simulink model "quadcopter_control_1"  (R2024b)
settings: Solver=ode45  StartTime=0.0  StopTime=10  RelTol=1e-3
libraries: slpidlib x6
settings Model: Creator=lenovo x390  LastModifiedBy=lenovo x390

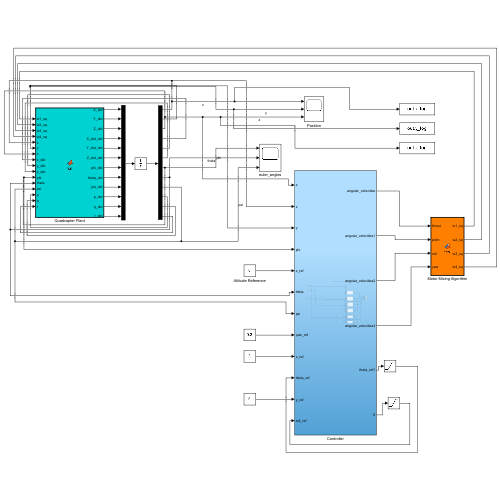
[thumbnail: Simulink's stored preview of the top-level diagram]
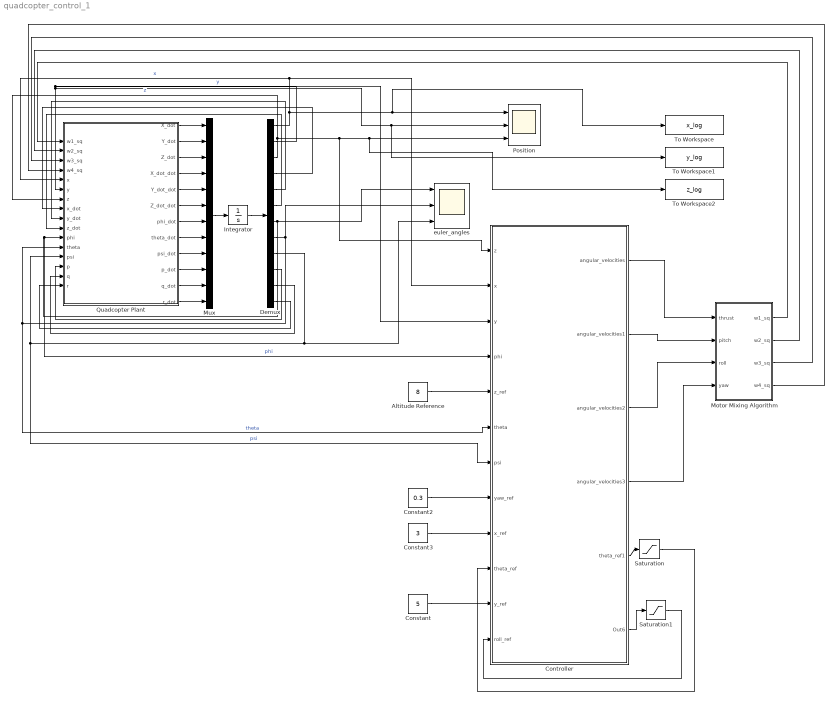
== system quadcopter_control_1 ==
  Altitude Reference : Constant  Value=8
  Constant : Constant  Value=5
  Constant2 : Constant  Value=0.3
  Constant3 : Constant  Value=3
  Controller : Subsystem
  Demux : Demux  Outputs=12
  Integrator : Integrator  InitialCondition=[0 0 1 0 0 0 0 0 0 0 0 0]
  Motor Mixing Algorithm : MATLAB Function  TreatAsAtomicUnit=on
  Mux : Mux  Inputs=12
  Position : Scope  NumInputPorts=3
  Quadcopter Plant : MATLAB Function  TreatAsAtomicUnit=on
  Saturation : Saturate
  Saturation1 : Saturate  UpperLimit=+0.3  LowerLimit=-0.3
  To Workspace : ToWorkspace  VariableName=x_log  SaveFormat=Timeseries  SampleTime=-1
  To Workspace1 : ToWorkspace  VariableName=y_log  SaveFormat=Timeseries  SampleTime=-1
  To Workspace2 : ToWorkspace  VariableName=z_log  SaveFormat=Timeseries  SampleTime=-1
  euler_angles : Scope  NumInputPorts=3
  wires:
  Quadcopter Plant/1(X_dot) -> Mux/1
  Quadcopter Plant/2(Y_dot) -> Mux/2
  Quadcopter Plant/3(Z_dot) -> Mux/3
  Quadcopter Plant/4(X_dot_dot) -> Mux/4
  Quadcopter Plant/5(Y_dot_dot) -> Mux/5
  Quadcopter Plant/6(Z_dot_dot) -> Mux/6
  Quadcopter Plant/7(phi_dot) -> Mux/7
  Quadcopter Plant/8(theta_dot) -> Mux/8
  Quadcopter Plant/9(psi_dot) -> Mux/9
  Quadcopter Plant/10(p_dot) -> Mux/10
  Quadcopter Plant/11(q_dot) -> Mux/11
  Quadcopter Plant/12(r_dot) -> Mux/12
  Mux/1 -> Integrator/1
  Integrator/1 -> Demux/1
  Demux/1 -> Quadcopter Plant/5(x), Controller/2(x), To Workspace/1, Position/1  "x"
  Demux/2 -> Quadcopter Plant/6(y), To Workspace1/1, Position/2, Controller/3(y)  "y"
  Demux/3 -> Quadcopter Plant/7(z), Controller/1(z), To Workspace2/1, Position/3  "z"
  Demux/4 -> Quadcopter Plant/8(x_dot)
  Demux/5 -> Quadcopter Plant/9(y_dot)
  Demux/6 -> Quadcopter Plant/10(z_dot)
  Demux/7 -> Controller/4(phi), Quadcopter Plant/11(phi), euler_angles/1  "phi"
  Demux/8 -> Controller/6(theta), Quadcopter Plant/12(theta), euler_angles/2  "theta"
  Demux/9 -> Controller/7(psi), Quadcopter Plant/13(psi), euler_angles/3  "psi"
  Demux/10 -> Quadcopter Plant/14(p)
  Demux/11 -> Quadcopter Plant/15(q)
  Demux/12 -> Quadcopter Plant/16(r)
  Motor Mixing Algorithm/1(w1_sq) -> Quadcopter Plant/1(w1_sq)
  Motor Mixing Algorithm/2(w2_sq) -> Quadcopter Plant/2(w2_sq)
  Motor Mixing Algorithm/3(w3_sq) -> Quadcopter Plant/3(w3_sq)
  Motor Mixing Algorithm/4(w4_sq) -> Quadcopter Plant/4(w4_sq)
  Altitude Reference/1 -> Controller/5(z_ref)
  Constant2/1 -> Controller/8(yaw_ref)
  Constant3/1 -> Controller/9(x_ref)
  Saturation/1 -> Controller/10(theta_ref)
  Constant/1 -> Controller/11(y_ref)
  Saturation1/1 -> Controller/12(roll_ref)
  Controller/1(angular_velocities) -> Motor Mixing Algorithm/1(thrust)
  Controller/2(angular_velocities1) -> Motor Mixing Algorithm/2(pitch)
  Controller/3(angular_velocities2) -> Motor Mixing Algorithm/3(roll)
  Controller/4(angular_velocities3) -> Motor Mixing Algorithm/4(yaw)
  Controller/5(theta_ref1) -> Saturation/1
  Controller/6(Out6) -> Saturation1/1

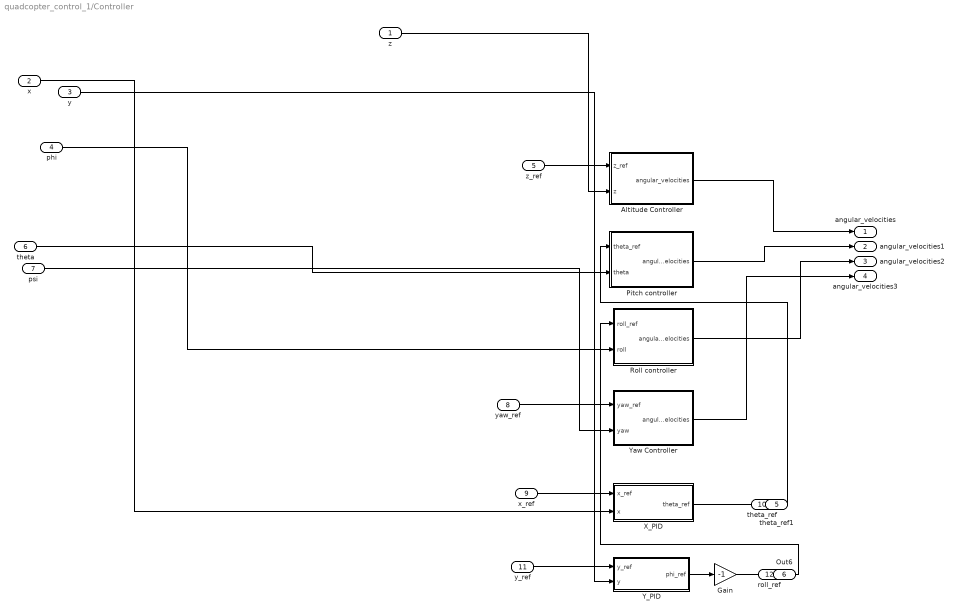
== system quadcopter_control_1/Controller ==
  z : Inport
  x : Inport  Port=2
  y : Inport  Port=3
  phi : Inport  Port=4
  z_ref : Inport  Port=5
  theta : Inport  Port=6
  psi : Inport  Port=7
  yaw_ref : Inport  Port=8
  x_ref : Inport  Port=9
  theta_ref : Inport  Port=10
  y_ref : Inport  Port=11
  roll_ref : Inport  Port=12
  Altitude Controller : Subsystem
  Gain : Gain  Gain=-1
  Pitch controller : Subsystem
  Roll controller : Subsystem
  X_PID : Subsystem
  Y_PID : Subsystem
  Yaw Controller : Subsystem
  angular_velocities : Outport
  angular_velocities1 : Outport  Port=2
  angular_velocities2 : Outport  Port=3
  angular_velocities3 : Outport  Port=4
  theta_ref1 : Outport  Port=5
  Out6 : Outport  Port=6
  wires:
  phi/1 -> Roll controller/2(roll)
  Pitch controller/1(angular_velocities) -> angular_velocities1/1
  theta/1 -> Pitch controller/2(theta)
  theta_ref/1 -> Pitch controller/1(theta_ref)
  Y_PID/1(phi_ref) -> Gain/1
  x/1 -> X_PID/2(x)
  Roll controller/1(angular_velocities) -> angular_velocities2/1
  Gain/1 -> Out6/1
  roll_ref/1 -> Roll controller/1(roll_ref)
  yaw_ref/1 -> Yaw Controller/1(yaw_ref)
  psi/1 -> Yaw Controller/2(yaw)
  x_ref/1 -> X_PID/1(x_ref)
  z_ref/1 -> Altitude Controller/1(z_ref)
  Yaw Controller/1(angular_velocities) -> angular_velocities3/1
  y/1 -> Y_PID/2(y)
  X_PID/1(theta_ref) -> theta_ref1/1
  z/1 -> Altitude Controller/2(z)
  Altitude Controller/1(angular_velocities) -> angular_velocities/1
  y_ref/1 -> Y_PID/1(y_ref)

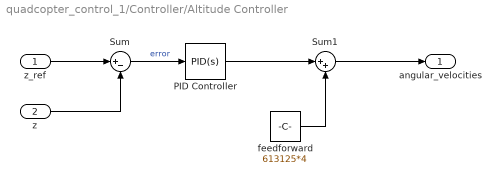
== system quadcopter_control_1/Controller/Altitude Controller ==
  z_ref : Inport
  z : Inport  Port=2
  PID Controller : slpidlib/PID Controller  Controller=PID  Form=Parallel  TimeDomain=Continuous-time  UseExternalTs=off  SampleTime=-1  IntegratorMethod=Forward Euler  FilterMethod=Forward Euler  ControllerParametersSource=internal  P=328860.941358092  I=45284.5767226925  UseKiTs=off  D=525153.531674945  UseExternalDerivativeSource=off  N=245.289249242135  UseFilter=on  TunerSelectOption=Transfer Function Based (PID Tuner App)  InitialConditionSource=internal  InitialConditionForIntegrator=0  InitialConditionForFilter=0  DifferentiatorICPrevScaledInput=0  ExternalReset=none  TrackingMode=off  Kt=1  LimitOutput=off  SatLimitsSource=internal  UpperSaturationLimit=inf  LowerSaturationLimit=-inf  LinearizeAsGain=on  AntiWindupMode=none  Kb=1  LimitIntegrator=off  UpperIntegratorSaturationLimit=inf  LowerIntegratorSaturationLimit=-inf  POutMin=[]  POutMax=[]  IOutMin=[]  IOutMax=[]  DOutMin=[]  DOutMax=[]  NOutMin=[]  NOutMax=[]  SumOutMin=[]  SumOutMax=[]  SaturationOutMin=[]  SaturationOutMax=[]  PParamMin=[]  PParamMax=[]  IParamMin=[]  IParamMax=[]  DParamMin=[]  DParamMax=[]  NParamMin=[]  NParamMax=[]  KbParamMin=[]  KbParamMax=[]  KtParamMin=[]  KtParamMax=[]  KbOutMin=[]  KbOutMax=[]  KtOutMin=[]  KtOutMax=[]  IntegratorOutMin=[]  IntegratorOutMax=[]  FilterOutMin=[]  FilterOutMax=[]  SumI1OutMin=[]  SumI1OutMax=[]  SumI2OutMin=[]  SumI2OutMax=[]  SumI3OutMin=[]  SumI3OutMax=[]  SumI4OutMin=[]  SumI4OutMax=[]  SumDOutMin=[]  SumDOutMax=[]  DifferentiatorOutMin=[]  DifferentiatorOutMax=[]  FilterDiffOutCoefMin=[]  FilterDiffOutCoefMax=[]  ReciprocalOutMin=[]  ReciprocalOutMax=[]  SumDenOutMin=[]  SumDenOutMax=[]  SumNumOutMin=[]  SumNumOutMax=[]  DivideOutMin=[]  DivideOutMax=[]  UdiffTsProdOutMin=[]  UdiffTsProdOutMax=[]  NTsProdOutMin=[]  NTsProdOutMax=[]  UintegralTsProdOutMin=[]  UintegralTsProdOutMax=[]  UngainTsProdOutMin=[]  UngainTsProdOutMax=[]  ClampingZeroOutDataTypeStr=Inherit: Inherit via back propagation  ClampingZeroOutMin=[]  ClampingZeroOutMax=[]  FilterDenConstantOutDataTypeStr=Inherit: Inherit via back propagation  FilterDenConstantOutMin=[]  FilterDenConstantOutMax=[]  PCopyOutDataTypeStr=Inherit: Inherit via back propagation  PCopyOutMin=[]  PCopyOutMax=[]  NCopyOutDataTypeStr=Inherit: Inherit via back propagation  NCopyOutMin=[]  NCopyOutMax=[]  IntegratorContinuousStateAttributes=''  IntegratorStateMustResolveToSignalObject=off  IntegratorRTWStateStorageClass=Auto  FilterContinuousStateAttributes=''  FilterStateMustResolveToSignalObject=off  FilterRTWStateStorageClass=Auto  ParallelPVariant=InternalParameters  IdealPVariant=Disabled  IVariant=InternalParameters  DVariant=InternalParameters  IntegratorVariant=Continuous  SatVariant=Disabled  AWVariant=Passthrough  PCopyVariant=Disabled  TRVariant=Disabled  FdbkBlocksVariant=Forward  IdealPFdbkVariant=Disabled  SatFdbkVariant=Disabled  DerivativeFilterVariant=ContFilter  NVariant=InternalParameters  NCopyVariant=Disabled  FilterICVariant=InternalICsFilter  IntegratorICVariant=InternalICs  ExternalResetVariant=Disabled  TRSumVariant=Passthrough  SumFdbkVariant=Disabled  SumVariant=Sum_PID  TsampFilterVariant=InternalTs  TsampNgainVariant=Passthrough  TsampIntegralVariant=Disabled_SignalSpec  ExternalSaturationOutDataTypeStr=Inherit: Same as second input  DerivativeSourceVariant=ErrorSignal  PreIntVariant=InternalPreInt
  Sum : Sum  Inputs=|+-
  Sum1 : Sum  Inputs=|++
  feedforward : Constant  Value=613125*4
  angular_velocities : Outport
  wires:
  z_ref/1 -> Sum/1
  Sum/1 -> PID Controller/1  "error"
  z/1 -> Sum/2
  PID Controller/1 -> Sum1/1
  Sum1/1 -> angular_velocities/1
  feedforward/1 -> Sum1/2

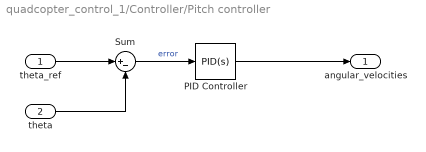
== system quadcopter_control_1/Controller/Pitch controller ==
  theta_ref : Inport
  theta : Inport  Port=2
  PID Controller : slpidlib/PID Controller  Controller=PID  Form=Parallel  TimeDomain=Continuous-time  UseExternalTs=off  SampleTime=-1  IntegratorMethod=Forward Euler  FilterMethod=Forward Euler  ControllerParametersSource=internal  P=-40128389715.2087  I=-9618985288819.15  UseKiTs=off  D=-38540591.5540109  UseExternalDerivativeSource=off  N=798113.129115548  UseFilter=on  TunerSelectOption=Transfer Function Based (PID Tuner App)  InitialConditionSource=internal  InitialConditionForIntegrator=0  InitialConditionForFilter=0  DifferentiatorICPrevScaledInput=0  ExternalReset=none  TrackingMode=off  Kt=1  LimitOutput=off  SatLimitsSource=internal  UpperSaturationLimit=inf  LowerSaturationLimit=-inf  LinearizeAsGain=on  AntiWindupMode=none  Kb=1  LimitIntegrator=off  UpperIntegratorSaturationLimit=inf  LowerIntegratorSaturationLimit=-inf  POutMin=[]  POutMax=[]  IOutMin=[]  IOutMax=[]  DOutMin=[]  DOutMax=[]  NOutMin=[]  NOutMax=[]  SumOutMin=[]  SumOutMax=[]  SaturationOutMin=[]  SaturationOutMax=[]  PParamMin=[]  PParamMax=[]  IParamMin=[]  IParamMax=[]  DParamMin=[]  DParamMax=[]  NParamMin=[]  NParamMax=[]  KbParamMin=[]  KbParamMax=[]  KtParamMin=[]  KtParamMax=[]  KbOutMin=[]  KbOutMax=[]  KtOutMin=[]  KtOutMax=[]  IntegratorOutMin=[]  IntegratorOutMax=[]  FilterOutMin=[]  FilterOutMax=[]  SumI1OutMin=[]  SumI1OutMax=[]  SumI2OutMin=[]  SumI2OutMax=[]  SumI3OutMin=[]  SumI3OutMax=[]  SumI4OutMin=[]  SumI4OutMax=[]  SumDOutMin=[]  SumDOutMax=[]  DifferentiatorOutMin=[]  DifferentiatorOutMax=[]  FilterDiffOutCoefMin=[]  FilterDiffOutCoefMax=[]  ReciprocalOutMin=[]  ReciprocalOutMax=[]  SumDenOutMin=[]  SumDenOutMax=[]  SumNumOutMin=[]  SumNumOutMax=[]  DivideOutMin=[]  DivideOutMax=[]  UdiffTsProdOutMin=[]  UdiffTsProdOutMax=[]  NTsProdOutMin=[]  NTsProdOutMax=[]  UintegralTsProdOutMin=[]  UintegralTsProdOutMax=[]  UngainTsProdOutMin=[]  UngainTsProdOutMax=[]  ClampingZeroOutDataTypeStr=Inherit: Inherit via back propagation  ClampingZeroOutMin=[]  ClampingZeroOutMax=[]  FilterDenConstantOutDataTypeStr=Inherit: Inherit via back propagation  FilterDenConstantOutMin=[]  FilterDenConstantOutMax=[]  PCopyOutDataTypeStr=Inherit: Inherit via back propagation  PCopyOutMin=[]  PCopyOutMax=[]  NCopyOutDataTypeStr=Inherit: Inherit via back propagation  NCopyOutMin=[]  NCopyOutMax=[]  IntegratorContinuousStateAttributes=''  IntegratorStateMustResolveToSignalObject=off  IntegratorRTWStateStorageClass=Auto  FilterContinuousStateAttributes=''  FilterStateMustResolveToSignalObject=off  FilterRTWStateStorageClass=Auto  ParallelPVariant=InternalParameters  IdealPVariant=Disabled  IVariant=InternalParameters  DVariant=InternalParameters  IntegratorVariant=Continuous  SatVariant=Disabled  AWVariant=Passthrough  PCopyVariant=Disabled  TRVariant=Disabled  FdbkBlocksVariant=Forward  IdealPFdbkVariant=Disabled  SatFdbkVariant=Disabled  DerivativeFilterVariant=ContFilter  NVariant=InternalParameters  NCopyVariant=Disabled  FilterICVariant=InternalICsFilter  IntegratorICVariant=InternalICs  ExternalResetVariant=Disabled  TRSumVariant=Passthrough  SumFdbkVariant=Disabled  SumVariant=Sum_PID  TsampFilterVariant=InternalTs  TsampNgainVariant=Passthrough  TsampIntegralVariant=Disabled_SignalSpec  ExternalSaturationOutDataTypeStr=Inherit: Same as second input  DerivativeSourceVariant=ErrorSignal  PreIntVariant=InternalPreInt
  Sum : Sum  Inputs=|+-
  angular_velocities : Outport
  wires:
  PID Controller/1 -> angular_velocities/1
  theta_ref/1 -> Sum/1
  Sum/1 -> PID Controller/1  "error"
  theta/1 -> Sum/2

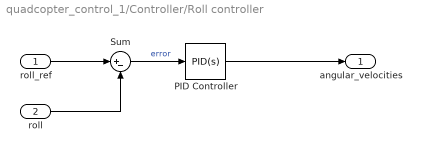
== system quadcopter_control_1/Controller/Roll controller ==
  roll_ref : Inport
  roll : Inport  Port=2
  PID Controller : slpidlib/PID Controller  Controller=PID  Form=Parallel  TimeDomain=Continuous-time  UseExternalTs=off  SampleTime=-1  IntegratorMethod=Forward Euler  FilterMethod=Forward Euler  ControllerParametersSource=internal  P=353723235658.445  I=209531659629859  UseKiTs=off  D=121145786.402814  UseExternalDerivativeSource=off  N=2506506.24433265  UseFilter=on  TunerSelectOption=Transfer Function Based (PID Tuner App)  InitialConditionSource=internal  InitialConditionForIntegrator=0  InitialConditionForFilter=0  DifferentiatorICPrevScaledInput=0  ExternalReset=none  TrackingMode=off  Kt=1  LimitOutput=off  SatLimitsSource=internal  UpperSaturationLimit=inf  LowerSaturationLimit=-inf  LinearizeAsGain=on  AntiWindupMode=none  Kb=1  LimitIntegrator=off  UpperIntegratorSaturationLimit=inf  LowerIntegratorSaturationLimit=-inf  POutMin=[]  POutMax=[]  IOutMin=[]  IOutMax=[]  DOutMin=[]  DOutMax=[]  NOutMin=[]  NOutMax=[]  SumOutMin=[]  SumOutMax=[]  SaturationOutMin=[]  SaturationOutMax=[]  PParamMin=[]  PParamMax=[]  IParamMin=[]  IParamMax=[]  DParamMin=[]  DParamMax=[]  NParamMin=[]  NParamMax=[]  KbParamMin=[]  KbParamMax=[]  KtParamMin=[]  KtParamMax=[]  KbOutMin=[]  KbOutMax=[]  KtOutMin=[]  KtOutMax=[]  IntegratorOutMin=[]  IntegratorOutMax=[]  FilterOutMin=[]  FilterOutMax=[]  SumI1OutMin=[]  SumI1OutMax=[]  SumI2OutMin=[]  SumI2OutMax=[]  SumI3OutMin=[]  SumI3OutMax=[]  SumI4OutMin=[]  SumI4OutMax=[]  SumDOutMin=[]  SumDOutMax=[]  DifferentiatorOutMin=[]  DifferentiatorOutMax=[]  FilterDiffOutCoefMin=[]  FilterDiffOutCoefMax=[]  ReciprocalOutMin=[]  ReciprocalOutMax=[]  SumDenOutMin=[]  SumDenOutMax=[]  SumNumOutMin=[]  SumNumOutMax=[]  DivideOutMin=[]  DivideOutMax=[]  UdiffTsProdOutMin=[]  UdiffTsProdOutMax=[]  NTsProdOutMin=[]  NTsProdOutMax=[]  UintegralTsProdOutMin=[]  UintegralTsProdOutMax=[]  UngainTsProdOutMin=[]  UngainTsProdOutMax=[]  ClampingZeroOutDataTypeStr=Inherit: Inherit via back propagation  ClampingZeroOutMin=[]  ClampingZeroOutMax=[]  FilterDenConstantOutDataTypeStr=Inherit: Inherit via back propagation  FilterDenConstantOutMin=[]  FilterDenConstantOutMax=[]  PCopyOutDataTypeStr=Inherit: Inherit via back propagation  PCopyOutMin=[]  PCopyOutMax=[]  NCopyOutDataTypeStr=Inherit: Inherit via back propagation  NCopyOutMin=[]  NCopyOutMax=[]  IntegratorContinuousStateAttributes=''  IntegratorStateMustResolveToSignalObject=off  IntegratorRTWStateStorageClass=Auto  FilterContinuousStateAttributes=''  FilterStateMustResolveToSignalObject=off  FilterRTWStateStorageClass=Auto  ParallelPVariant=InternalParameters  IdealPVariant=Disabled  IVariant=InternalParameters  DVariant=InternalParameters  IntegratorVariant=Continuous  SatVariant=Disabled  AWVariant=Passthrough  PCopyVariant=Disabled  TRVariant=Disabled  FdbkBlocksVariant=Forward  IdealPFdbkVariant=Disabled  SatFdbkVariant=Disabled  DerivativeFilterVariant=ContFilter  NVariant=InternalParameters  NCopyVariant=Disabled  FilterICVariant=InternalICsFilter  IntegratorICVariant=InternalICs  ExternalResetVariant=Disabled  TRSumVariant=Passthrough  SumFdbkVariant=Disabled  SumVariant=Sum_PID  TsampFilterVariant=InternalTs  TsampNgainVariant=Passthrough  TsampIntegralVariant=Disabled_SignalSpec  ExternalSaturationOutDataTypeStr=Inherit: Same as second input  DerivativeSourceVariant=ErrorSignal  PreIntVariant=InternalPreInt
  Sum : Sum  Inputs=|+-
  angular_velocities : Outport
  wires:
  roll/1 -> Sum/2
  PID Controller/1 -> angular_velocities/1
  Sum/1 -> PID Controller/1  "error"
  roll_ref/1 -> Sum/1

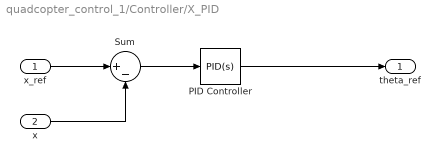
== system quadcopter_control_1/Controller/X_PID ==
  x_ref : Inport
  x : Inport  Port=2
  PID Controller : slpidlib/PID Controller  Controller=PID  Form=Parallel  TimeDomain=Continuous-time  UseExternalTs=off  SampleTime=-1  IntegratorMethod=Forward Euler  FilterMethod=Forward Euler  ControllerParametersSource=internal  P=0.000588535015865809  I=7.63170002463716e-05  UseKiTs=off  D=0.00109283634803694  UseExternalDerivativeSource=off  N=24.4449046575922  UseFilter=on  TunerSelectOption=Transfer Function Based (PID Tuner App)  InitialConditionSource=internal  InitialConditionForIntegrator=0  InitialConditionForFilter=0  DifferentiatorICPrevScaledInput=0  ExternalReset=none  TrackingMode=off  Kt=1  LimitOutput=off  SatLimitsSource=internal  UpperSaturationLimit=inf  LowerSaturationLimit=-inf  LinearizeAsGain=on  AntiWindupMode=none  Kb=1  LimitIntegrator=off  UpperIntegratorSaturationLimit=inf  LowerIntegratorSaturationLimit=-inf  POutMin=[]  POutMax=[]  IOutMin=[]  IOutMax=[]  DOutMin=[]  DOutMax=[]  NOutMin=[]  NOutMax=[]  SumOutMin=[]  SumOutMax=[]  SaturationOutMin=[]  SaturationOutMax=[]  PParamMin=[]  PParamMax=[]  IParamMin=[]  IParamMax=[]  DParamMin=[]  DParamMax=[]  NParamMin=[]  NParamMax=[]  KbParamMin=[]  KbParamMax=[]  KtParamMin=[]  KtParamMax=[]  KbOutMin=[]  KbOutMax=[]  KtOutMin=[]  KtOutMax=[]  IntegratorOutMin=[]  IntegratorOutMax=[]  FilterOutMin=[]  FilterOutMax=[]  SumI1OutMin=[]  SumI1OutMax=[]  SumI2OutMin=[]  SumI2OutMax=[]  SumI3OutMin=[]  SumI3OutMax=[]  SumI4OutMin=[]  SumI4OutMax=[]  SumDOutMin=[]  SumDOutMax=[]  DifferentiatorOutMin=[]  DifferentiatorOutMax=[]  FilterDiffOutCoefMin=[]  FilterDiffOutCoefMax=[]  ReciprocalOutMin=[]  ReciprocalOutMax=[]  SumDenOutMin=[]  SumDenOutMax=[]  SumNumOutMin=[]  SumNumOutMax=[]  DivideOutMin=[]  DivideOutMax=[]  UdiffTsProdOutMin=[]  UdiffTsProdOutMax=[]  NTsProdOutMin=[]  NTsProdOutMax=[]  UintegralTsProdOutMin=[]  UintegralTsProdOutMax=[]  UngainTsProdOutMin=[]  UngainTsProdOutMax=[]  ClampingZeroOutDataTypeStr=Inherit: Inherit via back propagation  ClampingZeroOutMin=[]  ClampingZeroOutMax=[]  FilterDenConstantOutDataTypeStr=Inherit: Inherit via back propagation  FilterDenConstantOutMin=[]  FilterDenConstantOutMax=[]  PCopyOutDataTypeStr=Inherit: Inherit via back propagation  PCopyOutMin=[]  PCopyOutMax=[]  NCopyOutDataTypeStr=Inherit: Inherit via back propagation  NCopyOutMin=[]  NCopyOutMax=[]  IntegratorContinuousStateAttributes=''  IntegratorStateMustResolveToSignalObject=off  IntegratorRTWStateStorageClass=Auto  FilterContinuousStateAttributes=''  FilterStateMustResolveToSignalObject=off  FilterRTWStateStorageClass=Auto  ParallelPVariant=InternalParameters  IdealPVariant=Disabled  IVariant=InternalParameters  DVariant=InternalParameters  IntegratorVariant=Continuous  SatVariant=Disabled  AWVariant=Passthrough  PCopyVariant=Disabled  TRVariant=Disabled  FdbkBlocksVariant=Forward  IdealPFdbkVariant=Disabled  SatFdbkVariant=Disabled  DerivativeFilterVariant=ContFilter  NVariant=InternalParameters  NCopyVariant=Disabled  FilterICVariant=InternalICsFilter  IntegratorICVariant=InternalICs  ExternalResetVariant=Disabled  TRSumVariant=Passthrough  SumFdbkVariant=Disabled  SumVariant=Sum_PID  TsampFilterVariant=InternalTs  TsampNgainVariant=Passthrough  TsampIntegralVariant=Disabled_SignalSpec  ExternalSaturationOutDataTypeStr=Inherit: Same as second input  DerivativeSourceVariant=ErrorSignal  PreIntVariant=InternalPreInt
  Sum : Sum  Inputs=|+-
  theta_ref : Outport
  wires:
  PID Controller/1 -> theta_ref/1
  x_ref/1 -> Sum/1
  Sum/1 -> PID Controller/1
  x/1 -> Sum/2

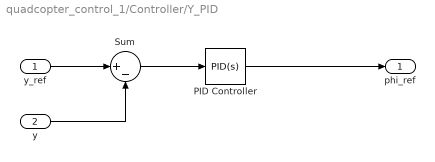
== system quadcopter_control_1/Controller/Y_PID ==
  y_ref : Inport
  y : Inport  Port=2
  PID Controller : slpidlib/PID Controller  Controller=PID  Form=Parallel  TimeDomain=Continuous-time  UseExternalTs=off  SampleTime=-1  IntegratorMethod=Forward Euler  FilterMethod=Forward Euler  ControllerParametersSource=internal  P=0.000622039047407379  I=8.48698303779395e-05  UseKiTs=off  D=0.00100064373755705  UseExternalDerivativeSource=off  N=242.610912674408  UseFilter=on  TunerSelectOption=Transfer Function Based (PID Tuner App)  InitialConditionSource=internal  InitialConditionForIntegrator=0  InitialConditionForFilter=0  DifferentiatorICPrevScaledInput=0  ExternalReset=none  TrackingMode=off  Kt=1  LimitOutput=off  SatLimitsSource=internal  UpperSaturationLimit=inf  LowerSaturationLimit=-inf  LinearizeAsGain=on  AntiWindupMode=none  Kb=1  LimitIntegrator=off  UpperIntegratorSaturationLimit=inf  LowerIntegratorSaturationLimit=-inf  POutMin=[]  POutMax=[]  IOutMin=[]  IOutMax=[]  DOutMin=[]  DOutMax=[]  NOutMin=[]  NOutMax=[]  SumOutMin=[]  SumOutMax=[]  SaturationOutMin=[]  SaturationOutMax=[]  PParamMin=[]  PParamMax=[]  IParamMin=[]  IParamMax=[]  DParamMin=[]  DParamMax=[]  NParamMin=[]  NParamMax=[]  KbParamMin=[]  KbParamMax=[]  KtParamMin=[]  KtParamMax=[]  KbOutMin=[]  KbOutMax=[]  KtOutMin=[]  KtOutMax=[]  IntegratorOutMin=[]  IntegratorOutMax=[]  FilterOutMin=[]  FilterOutMax=[]  SumI1OutMin=[]  SumI1OutMax=[]  SumI2OutMin=[]  SumI2OutMax=[]  SumI3OutMin=[]  SumI3OutMax=[]  SumI4OutMin=[]  SumI4OutMax=[]  SumDOutMin=[]  SumDOutMax=[]  DifferentiatorOutMin=[]  DifferentiatorOutMax=[]  FilterDiffOutCoefMin=[]  FilterDiffOutCoefMax=[]  ReciprocalOutMin=[]  ReciprocalOutMax=[]  SumDenOutMin=[]  SumDenOutMax=[]  SumNumOutMin=[]  SumNumOutMax=[]  DivideOutMin=[]  DivideOutMax=[]  UdiffTsProdOutMin=[]  UdiffTsProdOutMax=[]  NTsProdOutMin=[]  NTsProdOutMax=[]  UintegralTsProdOutMin=[]  UintegralTsProdOutMax=[]  UngainTsProdOutMin=[]  UngainTsProdOutMax=[]  ClampingZeroOutDataTypeStr=Inherit: Inherit via back propagation  ClampingZeroOutMin=[]  ClampingZeroOutMax=[]  FilterDenConstantOutDataTypeStr=Inherit: Inherit via back propagation  FilterDenConstantOutMin=[]  FilterDenConstantOutMax=[]  PCopyOutDataTypeStr=Inherit: Inherit via back propagation  PCopyOutMin=[]  PCopyOutMax=[]  NCopyOutDataTypeStr=Inherit: Inherit via back propagation  NCopyOutMin=[]  NCopyOutMax=[]  IntegratorContinuousStateAttributes=''  IntegratorStateMustResolveToSignalObject=off  IntegratorRTWStateStorageClass=Auto  FilterContinuousStateAttributes=''  FilterStateMustResolveToSignalObject=off  FilterRTWStateStorageClass=Auto  ParallelPVariant=InternalParameters  IdealPVariant=Disabled  IVariant=InternalParameters  DVariant=InternalParameters  IntegratorVariant=Continuous  SatVariant=Disabled  AWVariant=Passthrough  PCopyVariant=Disabled  TRVariant=Disabled  FdbkBlocksVariant=Forward  IdealPFdbkVariant=Disabled  SatFdbkVariant=Disabled  DerivativeFilterVariant=ContFilter  NVariant=InternalParameters  NCopyVariant=Disabled  FilterICVariant=InternalICsFilter  IntegratorICVariant=InternalICs  ExternalResetVariant=Disabled  TRSumVariant=Passthrough  SumFdbkVariant=Disabled  SumVariant=Sum_PID  TsampFilterVariant=InternalTs  TsampNgainVariant=Passthrough  TsampIntegralVariant=Disabled_SignalSpec  ExternalSaturationOutDataTypeStr=Inherit: Same as second input  DerivativeSourceVariant=ErrorSignal  PreIntVariant=InternalPreInt
  Sum : Sum  Inputs=|+-
  phi_ref : Outport
  wires:
  y/1 -> Sum/2
  y_ref/1 -> Sum/1
  PID Controller/1 -> phi_ref/1
  Sum/1 -> PID Controller/1

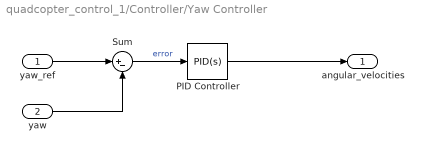
== system quadcopter_control_1/Controller/Yaw Controller ==
  yaw_ref : Inport
  yaw : Inport  Port=2
  PID Controller : slpidlib/PID Controller  Controller=PID  Form=Parallel  TimeDomain=Continuous-time  UseExternalTs=off  SampleTime=-1  IntegratorMethod=Forward Euler  FilterMethod=Forward Euler  ControllerParametersSource=internal  P=-191294.890855896  I=-49644.7720645806  UseKiTs=off  D=-169454.301661052  UseExternalDerivativeSource=off  N=866.923674741149  UseFilter=on  TunerSelectOption=Transfer Function Based (PID Tuner App)  InitialConditionSource=internal  InitialConditionForIntegrator=0  InitialConditionForFilter=0  DifferentiatorICPrevScaledInput=0  ExternalReset=none  TrackingMode=off  Kt=1  LimitOutput=off  SatLimitsSource=internal  UpperSaturationLimit=inf  LowerSaturationLimit=-inf  LinearizeAsGain=on  AntiWindupMode=none  Kb=1  LimitIntegrator=off  UpperIntegratorSaturationLimit=inf  LowerIntegratorSaturationLimit=-inf  POutMin=[]  POutMax=[]  IOutMin=[]  IOutMax=[]  DOutMin=[]  DOutMax=[]  NOutMin=[]  NOutMax=[]  SumOutMin=[]  SumOutMax=[]  SaturationOutMin=[]  SaturationOutMax=[]  PParamMin=[]  PParamMax=[]  IParamMin=[]  IParamMax=[]  DParamMin=[]  DParamMax=[]  NParamMin=[]  NParamMax=[]  KbParamMin=[]  KbParamMax=[]  KtParamMin=[]  KtParamMax=[]  KbOutMin=[]  KbOutMax=[]  KtOutMin=[]  KtOutMax=[]  IntegratorOutMin=[]  IntegratorOutMax=[]  FilterOutMin=[]  FilterOutMax=[]  SumI1OutMin=[]  SumI1OutMax=[]  SumI2OutMin=[]  SumI2OutMax=[]  SumI3OutMin=[]  SumI3OutMax=[]  SumI4OutMin=[]  SumI4OutMax=[]  SumDOutMin=[]  SumDOutMax=[]  DifferentiatorOutMin=[]  DifferentiatorOutMax=[]  FilterDiffOutCoefMin=[]  FilterDiffOutCoefMax=[]  ReciprocalOutMin=[]  ReciprocalOutMax=[]  SumDenOutMin=[]  SumDenOutMax=[]  SumNumOutMin=[]  SumNumOutMax=[]  DivideOutMin=[]  DivideOutMax=[]  UdiffTsProdOutMin=[]  UdiffTsProdOutMax=[]  NTsProdOutMin=[]  NTsProdOutMax=[]  UintegralTsProdOutMin=[]  UintegralTsProdOutMax=[]  UngainTsProdOutMin=[]  UngainTsProdOutMax=[]  ClampingZeroOutDataTypeStr=Inherit: Inherit via back propagation  ClampingZeroOutMin=[]  ClampingZeroOutMax=[]  FilterDenConstantOutDataTypeStr=Inherit: Inherit via back propagation  FilterDenConstantOutMin=[]  FilterDenConstantOutMax=[]  PCopyOutDataTypeStr=Inherit: Inherit via back propagation  PCopyOutMin=[]  PCopyOutMax=[]  NCopyOutDataTypeStr=Inherit: Inherit via back propagation  NCopyOutMin=[]  NCopyOutMax=[]  IntegratorContinuousStateAttributes=''  IntegratorStateMustResolveToSignalObject=off  IntegratorRTWStateStorageClass=Auto  FilterContinuousStateAttributes=''  FilterStateMustResolveToSignalObject=off  FilterRTWStateStorageClass=Auto  ParallelPVariant=InternalParameters  IdealPVariant=Disabled  IVariant=InternalParameters  DVariant=InternalParameters  IntegratorVariant=Continuous  SatVariant=Disabled  AWVariant=Passthrough  PCopyVariant=Disabled  TRVariant=Disabled  FdbkBlocksVariant=Forward  IdealPFdbkVariant=Disabled  SatFdbkVariant=Disabled  DerivativeFilterVariant=ContFilter  NVariant=InternalParameters  NCopyVariant=Disabled  FilterICVariant=InternalICsFilter  IntegratorICVariant=InternalICs  ExternalResetVariant=Disabled  TRSumVariant=Passthrough  SumFdbkVariant=Disabled  SumVariant=Sum_PID  TsampFilterVariant=InternalTs  TsampNgainVariant=Passthrough  TsampIntegralVariant=Disabled_SignalSpec  ExternalSaturationOutDataTypeStr=Inherit: Same as second input  DerivativeSourceVariant=ErrorSignal  PreIntVariant=InternalPreInt
  Sum : Sum  Inputs=|+-
  angular_velocities : Outport
  wires:
  yaw_ref/1 -> Sum/1
  yaw/1 -> Sum/2
  PID Controller/1 -> angular_velocities/1
  Sum/1 -> PID Controller/1  "error"

== matlab function quadcopter_control_1/Motor Mixing Algorithm ==
  data: thrust input; w1_sq output; pitch input; roll input; yaw input; w2_sq output; w3_sq output; w4_sq output
function[w1_sq,w2_sq,w3_sq,w4_sq]= fcn(thrust,pitch,roll,yaw)
thrust=0.25*thrust;
w1_sq = thrust + roll - yaw;
w2_sq = thrust - pitch + yaw;
w3_sq = thrust - roll - yaw;
w4_sq = thrust + pitch + yaw;

== matlab function quadcopter_control_1/Quadcopter Plant ==
  data: X_dot output; Y_dot output; w1_sq input; w2_sq input; w3_sq input; w4_sq input; x input; y input; z input; x_dot input; y_dot input; z_dot input; phi input; theta input; psi input; p input; q input; r input; Z_dot output; X_dot_dot output; Y_dot_dot output; Z_dot_dot output; phi_dot output; theta_dot output; psi_dot output; p_dot output; q_dot output; r_dot output
function [X_dot,Y_dot,Z_dot,X_dot_dot,Y_dot_dot,Z_dot_dot,...
          phi_dot,theta_dot,psi_dot,p_dot,q_dot,r_dot] = ...
          fcn(w1_sq,w2_sq,w3_sq,w4_sq,x,y,z,x_dot,y_dot,z_dot,phi,theta,psi,p,q,r)

% Physical parameters
m   = 0.5;
g   = 9.81;
L   = 0.225;
I_xx = 5.0e-3;
I_yy = 5.0e-3;
I_zz = 9.0e-3;
k   = 2.0e-6;
b   = 1.0e-7;
k_D = 0.1;

% Rotation matrix
R = [cos(theta)*cos(psi), sin(phi)*sin(theta)*cos(psi) - cos(phi)*sin(psi), cos(phi)*sin(theta)*cos(psi) + sin(phi)*sin(psi);
     cos(theta)*sin(psi), sin(phi)*sin(theta)*sin(psi) + cos(phi)*cos(psi), cos(phi)*sin(theta)*sin(psi) - sin(phi)*cos(psi);
     -sin(theta),         sin(phi)*cos(theta),                              cos(phi)*cos(theta)];

% Thrust vector (body frame)
Tb = [0; 0; k*(w1_sq+w2_sq+w3_sq+w4_sq)];
%simulating a roll
%delta=10000;
%w1_sq=w1_sq+delta;
%w3_sq=w3_sq-delta;
% Drag force (inertial frame)
Fd = -k_D * [x_dot; y_dot; z_dot];

% Linear accelerations
acc = (1/m)*(R*Tb + Fd) + [0; 0; -g];
X_dot_dot = acc(1);
Y_dot_dot = acc(2);
Z_dot_dot = acc(3);

% Position rates (trivial)
X_dot = x_dot;
Y_dot = y_dot;
Z_dot = z_dot;

% Euler angle rates
phi_dot   = p + q*sin(phi)*tan(theta) + r*cos(phi)*tan(theta);
theta_dot = q*cos(phi) - r*sin(phi);
psi_dot   = q*(sin(phi)/cos(theta)) + r*(cos(phi)/cos(theta));

% Torque vector
tau = [L*k*(w1_sq - w3_sq);
       L*k*(w2_sq - w4_sq);
       b*(w1_sq - w2_sq + w3_sq - w4_sq)];

% Angular acceleration
p_dot = (tau(1) - (I_zz-I_yy)*q*r) / I_xx;
q_dot = (tau(2) - (I_xx-I_zz)*p*r) / I_yy;
r_dot = (tau(3) - (I_yy-I_xx)*p*q) / I_zz;
